simulink model "r2_2f_4x_4a_4k_r366"  (R2012b)
(part 4 of 114)

  [vacc_txeof2] -> Concat6/1
  fake_vacc2/5(pkt_rdy) -> [vacc_ready2]
  fake_vacc3/5(pkt_rdy) -> [vacc_ready3]
  bus_expand1/1(msb_out2) -> [go2]
  bus_expand1/2(lsb_out1) -> [go3]
  [vacc_ready2] -> Concat7/1
  [vacc_ready3] -> Concat7/2
  [id3] -> pre_process3/9(board_id)
  ctrl/7(in_loopback_rst) -> edge_detect1/1(in)
  ctrl/1(in_rst) -> pipeline/1(d)
  ctrl/6(in_leds_en) -> pipeline8/1(d)
  ctrl/5(in_comms_en) -> pipeline5/1(d)
  ctrl/2(in_status_clr) -> edge_detect/1(in)
  ctrl/4(in_comms_status_clr) -> edge_detect2/1(in)
  ctrl/3(in_comms_rst) -> pipeline6/1(d)
  gbe_mux_bus1/1(input) -> Terminator10/1
  gbe_mux_bus1/2(do) -> [gbe_txd1]
  gbe_mux_bus1/3(valido) -> [gbe_txvld1]
  gbe_mux_bus1/4(eofo) -> [gbe_txeof1]
  gbe_mux_bus1/5(start) -> bus_expand1/1(bus_in)
  Concat4/1 -> gbe_mux_bus1/1(di)
  Concat5/1 -> gbe_mux_bus1/2(validi)
  Concat6/1 -> gbe_mux_bus1/3(eofi)
  Concat7/1 -> gbe_mux_bus1/4(drdy)
  [go0] -> pack_out0/3(pkt_rdy)
  Delay23/1(q) -> [vacc_txd0]
  board_id/1(in_reg) -> Concat8/1
  Constant21/1 -> Concat8/2
  Concat8/1 -> Delay72/1(d)
  [gbe_out_en] -> Register/1
  Register/1 -> Logical/1
  pack_out0/2(valid_out) -> Delay5/1(d)
  Logical/1 -> [vacc_txvld0]
  pack_out1/2(valid_out) -> Delay1/1(d)
  Delay5/1(q) -> Logical/2
  pack_out3/2(valid_out) -> Delay8/1(d)
  pack_out2/2(valid_out) -> Delay13/1(d)
  Delay3/1(q) -> [vacc_txeof1], Register1/2, vacc_monitor3/2(eof)
  [gbe_out_en] -> Register1/1
  Register1/1 -> Logical1/1
  Delay1/1(q) -> Logical1/2
  [go1] -> pack_out1/3(pkt_rdy)
  [go2] -> pack_out2/3(pkt_rdy)
  Delay47/1(q) -> vacc_monitor6/2(eof), [vacc_txeof2], Register2/2
  [gbe_out_en] -> Register2/1
  Register2/1 -> Logical12/1
  Delay13/1(q) -> Logical12/2
  Delay67/1(q) -> [vacc_txd2]
  Logical12/1 -> [vacc_txvld2]
  Delay76/1(q) -> vacc_monitor7/2(eof), [vacc_txeof3], Register3/2
  [gbe_out_en] -> Register3/1
  Register3/1 -> Logical13/1
  Delay8/1(q) -> Logical13/2
  [go3] -> pack_out3/3(pkt_rdy)
  Constant22/1 -> Relational16/1
  Relational16/1 -> Logical28/2
  Logical28/1 -> [valid_data_in0]
  pkt_reord_devel1/3(valid_out) -> delay11/1, snap_reord1/3(in_valid), snap_reord1/10(we), Logical3/2, Logical29/1, Delay11/1(d)
  pkt_reord_devel1/6(flag_out) -> Relational17/2, Slice4/1, Slice5/1, Slice6/1, Slice7/1
  Constant23/1 -> Relational17/1
  Relational17/1 -> Logical29/2
  Logical29/1 -> [valid_data_in1]
  pkt_reord_devel2/6(flag_out) -> Relational18/2, Slice27/1, Slice26/1, Slice23/1, Slice22/1
  Constant24/1 -> Relational18/1
  Relational18/1 -> Logical30/2
  Logical30/1 -> [valid_data_in2]
  pkt_reord_devel3/6(flag_out) -> Relational19/2, Slice36/1, Slice35/1, Slice34/1, Slice33/1
  Constant25/1 -> Relational19/1
  Relational19/1 -> Logical31/2
  Logical31/1 -> [valid_data_in3]
  latch3/15(rx_reg) -> status3/15(out_rxing_data)
  latch3/16(tx_reg) -> status3/16(out_txing_data)
  [valid_data_in3] -> latch3/16(rx)
  [accumulating3] -> latch3/17(tx)
  latch2/3(Out3) -> status2/3(out_feng_rx_err)
  latch2/2(Out2) -> status2/2(out_rx_dest_err)
  latch2/1(Out1) -> status2/1(out_gbe_down)
  [clr_status] -> latch2/1(reset)
  Inverter2/1 -> latch2/2(gbe_down)
  [gbe_rx_bad1] -> latch2/12(rx_bad_frame)
  [pre_adc_err2] -> latch2/8(adc_over)
  [gbe_tx_over1] -> latch2/13(tx_over)
  [pre_rx_dest_err2] -> latch2/3(rx_dest_err)
  [pre_ndiode_en2] -> latch2/9(noise_diode_en)
  [pre_feng_qdr_err2] -> latch2/6(feng_qdr_err)
  [xeng_rx_err2] -> latch2/14(xeng_bad_dat)
  [valid_data_in2] -> latch2/16(rx)
  [pre_fft_err2] -> latch2/5(fft_err)
  [vacc_err2] -> latch2/10(vacc_err)
  [pre_spead_err2] -> latch2/11(rx_bad_pkt)
  [pack_err2] -> latch2/15(pack_err)
  [pre_feng_rx_err2] -> latch2/4(feng_rx_err)
  [accumulating2] -> latch2/17(tx)
  [pre_feng_chk_err2] -> latch2/7(feng_chk_err)
  latch2/16(tx_reg) -> status2/16(out_txing_data)
  latch2/15(rx_reg) -> status2/15(out_rxing_data)
  latch2/12(Out12) -> status2/12(out_tx_over)
  latch2/6(Out6) -> status2/6(out_feng_chk_err)
  latch2/14(Out14) -> status2/14(out_pack_err)
  latch2/10(Out10) -> status2/10(out_rx_bad_pkt)
  latch2/7(Out7) -> status2/7(out_adc_over)
  latch2/9(Out9) -> status2/9(out_vacc_err)
  latch2/4(Out4) -> status2/4(out_fft_err)
  latch2/11(Out11) -> status2/11(out_rx_bad_frame)
  latch2/5(Out5) -> status2/5(out_feng_qdr_err)
  latch2/8(Out8) -> status2/8(out_noise_diode_en)
  latch2/13(Out13) -> status2/13(out_xeng_bad_dat)
  latch1/3(Out3) -> status1/3(out_feng_rx_err)
  latch1/2(Out2) -> status1/2(out_rx_dest_err)
  latch1/1(Out1) -> status1/1(out_gbe_down)
  latch1/16(tx_reg) -> status1/16(out_txing_data)
  latch1/15(rx_reg) -> status1/15(out_rxing_data)
  latch1/12(Out12) -> status1/12(out_tx_over)
  latch1/6(Out6) -> status1/6(out_feng_chk_err)
  latch1/14(Out14) -> status1/14(out_pack_err)
  latch1/10(Out10) -> status1/10(out_rx_bad_pkt)
  latch1/7(Out7) -> status1/7(out_adc_over)
  latch1/9(Out9) -> status1/9(out_vacc_err)
  latch1/4(Out4) -> status1/4(out_fft_err)
  latch1/11(Out11) -> status1/11(out_rx_bad_frame)
  latch1/5(Out5) -> status1/5(out_feng_qdr_err)
  latch1/8(Out8) -> status1/8(out_noise_diode_en)
  latch1/13(Out13) -> status1/13(out_xeng_bad_dat)
  [valid_data_in1] -> latch1/16(rx)
  [accumulating1] -> latch1/17(tx)
  latch1/17(data_bad) -> [data_in_bad1]
  latch1/18(error) -> [err1]
  latch1/19(flags) -> [flags1]
  [gbe_up0] -> Inverter6/1
  [clr_status] -> latch1/1(reset)
  [pack_err1] -> latch1/15(pack_err)
  [pre_rx_dest_err1] -> latch1/3(rx_dest_err)
  [pre_feng_rx_err1] -> latch1/4(feng_rx_err)
  [pre_ndiode_en1] -> latch1/9(noise_diode_en)
  [pre_adc_err1] -> latch1/8(adc_over)
  [vacc_err1] -> latch1/10(vacc_err)
  [pre_spead_err1] -> latch1/11(rx_bad_pkt)
  [pre_feng_chk_err1] -> latch1/7(feng_chk_err)
  [gbe_rx_bad0] -> latch1/12(rx_bad_frame)
  [pre_feng_qdr_err1] -> latch1/6(feng_qdr_err)
  [gbe_tx_over0] -> latch1/13(tx_over)
  [pre_fft_err1] -> latch1/5(fft_err)
  [xeng_rx_err1] -> latch1/14(xeng_bad_dat)
  Inverter6/1 -> latch1/2(gbe_down)
  latch0/3(Out3) -> status0/3(out_feng_rx_err)
  latch0/2(Out2) -> status0/2(out_rx_dest_err)
  latch0/1(Out1) -> status0/1(out_gbe_down)
  latch0/16(tx_reg) -> status0/16(out_txing_data)
  latch0/15(rx_reg) -> status0/15(out_rxing_data)
  latch0/12(Out12) -> status0/12(out_tx_over)
  latch0/6(Out6) -> status0/6(out_feng_chk_err)
  latch0/14(Out14) -> status0/14(out_pack_err)
  latch0/10(Out10) -> status0/10(out_rx_bad_pkt)
  latch0/7(Out7) -> status0/7(out_adc_over)
  latch0/9(Out9) -> status0/9(out_vacc_err)
  latch0/4(Out4) -> status0/4(out_fft_err)
  latch0/11(Out11) -> status0/11(out_rx_bad_frame)
  latch0/5(Out5) -> status0/5(out_feng_qdr_err)
  latch0/8(Out8) -> status0/8(out_noise_diode_en)
  latch0/13(Out13) -> status0/13(out_xeng_bad_dat)
  latch0/17(data_bad) -> [data_in_bad0]
  latch0/18(error) -> [err0]
  latch0/19(flags) -> [flags0]
  [gbe_up0] -> Inverter5/1
  [clr_status] -> latch0/1(reset)
  [pack_err0] -> latch0/15(pack_err)
  [pre_rx_dest_err0] -> latch0/3(rx_dest_err)
  [pre_feng_rx_err0] -> latch0/4(feng_rx_err)
  [pre_ndiode_en0] -> latch0/9(noise_diode_en)
  [pre_adc_err0] -> latch0/8(adc_over)
  [vacc_err0] -> latch0/10(vacc_err)
  [pre_spead_err0] -> latch0/11(rx_bad_pkt)
  [pre_feng_chk_err0] -> latch0/7(feng_chk_err)
  [gbe_rx_bad0] -> latch0/12(rx_bad_frame)
  [pre_feng_qdr_err0] -> latch0/6(feng_qdr_err)
  [gbe_tx_over0] -> latch0/13(tx_over)
  [pre_fft_err0] -> latch0/5(fft_err)
  [xeng_rx_err0] -> latch0/14(xeng_bad_dat)
  Inverter5/1 -> latch0/2(gbe_down)
  [valid_data_in0] -> latch0/16(rx)
  [accumulating0] -> latch0/17(tx)
  Delay30/1(q) -> snap_xeng0/3(trig), vacc_tvg0/2(sync_in)
  Delay31/1(q) -> 16b_32b/1(In1)
  Delay45/1(q) -> [accumulating0], snap_xeng0/2(we), vacc_tvg0/4(valid_in)
  Delay46/1(q) -> delay5/1
  Delay16/1(q) -> snap_xeng1/3(trig), vacc_tvg1/2(sync_in)
  Delay49/1(q) -> 16b_32b1/1(In1)
  Delay77/1(q) -> [accumulating1], snap_xeng1/2(we), vacc_tvg1/4(valid_in)
  Delay78/1(q) -> delay8/1
  Delay92/1(q) -> vacc_tvg2/2(sync_in), snap_xeng2/3(trig)
  Delay93/1(q) -> 16b_32b2/1(In1)
  Delay94/1(q) -> vacc_tvg2/4(valid_in), [accumulating2], snap_xeng2/2(we)
  Delay113/1(q) -> delay75/1
  Delay114/1(q) -> snap_xeng3/3(trig), vacc_tvg3/2(sync_in)
  Delay115/1(q) -> 16b_32b3/1(In1)
  Delay116/1(q) -> [accumulating3], snap_xeng3/2(we), vacc_tvg3/4(valid_in)
  Delay117/1(q) -> delay91/1
